simulink model "controller"  (Simulink 7.3)
settings: Solver=FixedStepDiscrete  StartTime=0.0  StopTime=inf  FixedStep=120  RelTol=1e-3
libraries: simulink x6
settings Model: Creator=mwetter  LastModifiedBy=mwetter

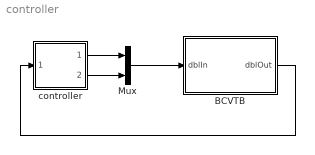
== system controller ==
  BCVTB : Subsystem  Description=Block that interfaces to the BCVTB.
  Mux : Mux  Inputs=2
  controller : Subsystem
  wires:
  controller/2(TSet) -> Mux/2
  controller/1(yHea) -> Mux/1
  Mux/1 -> BCVTB/1(dblIn)
  BCVTB/1(dblOut) -> controller/1(TMea)

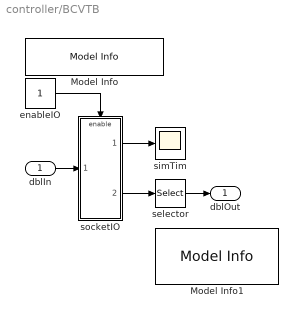
== system controller/BCVTB ==
  dblIn : Inport
  Model Info : simulink/Model-Wide Utilities/Model Info  SystemSampleTime=-1  InitialBlockCM=None  BlockCM=None  Frame=off  DisplayStringWithTags=%<Description>Set to 1 to enable I/O  HorizontalTextAlignment=Left  LeftAlignmentValue=0.02  SourceBlockDiagram=controller  TagMaxNumber=20
  Model Info1 : simulink/Model-Wide Utilities/Model Info  SystemSampleTime=-1  InitialBlockCM=None  BlockCM=None  Frame=off  DisplayStringWithTags=|  HorizontalTextAlignment=Left  LeftAlignmentValue=0.02  SourceBlockDiagram=controller  TagMaxNumber=20
      | The selector block selects 
      | a subset of the vector u 
      | and outputs it as the vector v.
  enableIO : Constant  OutDataType=sfix(16)  OutScaling=2^0
  selector : Selector  InputPortWidth=128  IndexOptions=Index vector (dialog)  Indices=[1]  OutputSizes=1
  simTim : Scope
  socketIO : Subsystem
  dblOut : Outport
  wires:
  selector/1 -> dblOut/1
  dblIn/1 -> socketIO/1(dblIn)
  socketIO/2(dblOut) -> selector/1
  enableIO/1 -> socketIO/Enable
  socketIO/1(simTim) -> simTim/1

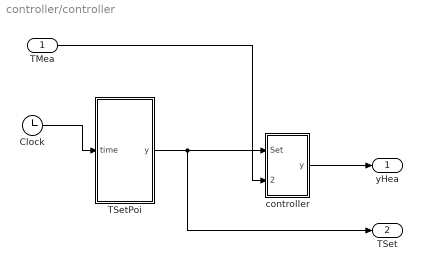
== system controller/controller ==
  TMea : Inport
  Clock : Clock
      settings: Decimation=10
  TSetPoi : Subsystem
  controller : Subsystem
  yHea : Outport
  TSet : Outport  Port=2
  wires:
  TSetPoi/1(y) -> controller/1(Set), TSet/1
  Clock/1 -> TSetPoi/1(time)
  TMea/1 -> controller/2(Mea)
  controller/1(y) -> yHea/1

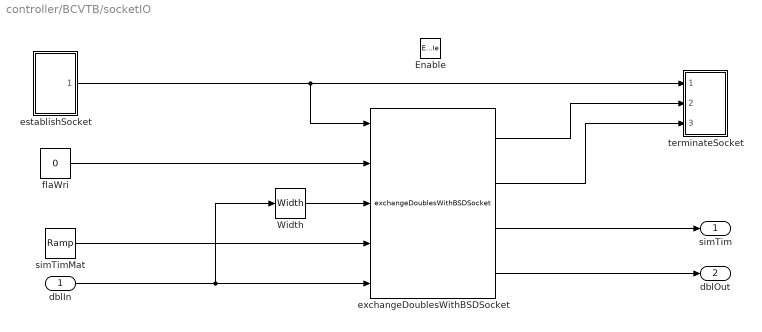
== system controller/BCVTB/socketIO ==
  dblIn : Inport
  Enable : EnablePort
  Width : Width  DataType=int16
  establishSocket : Subsystem  TreatAsAtomicUnit=on
  exchangeDoublesWithBSDSocket : S-Function  FunctionName=exchangeDoublesWithBSDSocket  EnableBusSupport=off  mask(Legacy Function){SFunctionSpec=int16 y1 = exchangeDoublesWithBSDSocket(int16 u1[1], int16 u2[1], int16 y2[1], double u3[1], double u4[], double y3[1], double y4[50]), ShowSpec=off}
      mask prompts: ShowSpec "Display function specification"
      mask help:
      | This block allows the user to call the following C function(s) in Simulink:
      |
      |  InitializeConditionsFcn: none
      |
      |  StartFcn: none
      |
      |  OutputFcn: int16 y1 = exchangeDoublesWithBSDSocket(int16 u1[1], int16 u2[1], int16 y2[1], double u3[1], double u4[], double y3[1], double y4[50])
      |
      |  TerminateFcn: none
      mask CallbackString:
      | |if strcmp(get_param(gcbh, 'ShowSpec'), 'on')
      |   set_param(gcbh, 'MaskDisplay', sprintf('fprintf(''%s'');', get_param(gcbh, 'SFunctionSpec')));
      | else
      |   set_param(gcbh, 'MaskDisplay', sprintf('fprintf(''%s'');', get_param(gcbh, 'FunctionName')));
      | end
      mask Display: fprintf('exchangeDoublesWithBSDSocket');
  flaWri : Constant  Value=0  OutDataTypeMode=int16  OutDataType=sfix(16)  OutScaling=2^0  OutDataTypeStr=int16
  simTimMat : simulink/Sources/Ramp  SystemSampleTime=-1  slope=1  start=0  X0=0
  terminateSocket : Subsystem
  simTim : Outport
  dblOut : Outport  Port=2
  wires:
  exchangeDoublesWithBSDSocket/2 -> terminateSocket/3(excFlaRea)
  exchangeDoublesWithBSDSocket/1 -> terminateSocket/2(excRetVal)
  exchangeDoublesWithBSDSocket/4 -> dblOut/1
  Width/1 -> exchangeDoublesWithBSDSocket/3
  simTimMat/1 -> exchangeDoublesWithBSDSocket/4
  dblIn/1 -> Width/1, exchangeDoublesWithBSDSocket/5
  exchangeDoublesWithBSDSocket/3 -> simTim/1
  flaWri/1 -> exchangeDoublesWithBSDSocket/2
  establishSocket/1(socketFD) -> terminateSocket/1(sockfd), exchangeDoublesWithBSDSocket/1

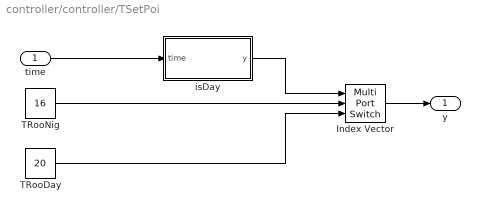
== system controller/controller/TSetPoi ==
  time : Inport  OutDataType=sfix(16)  OutScaling=2^0
  Index Vector : MultiPortSwitch  Inputs=2  zeroidx=on  OutDataType=sfix(16)  OutScaling=2^0
  TRooDay : Constant  Value=20  OutDataType=sfix(16)  OutScaling=2^0
  TRooNig : Constant  Value=16  OutDataType=sfix(16)  OutScaling=2^0
  isDay : Subsystem
  y : Outport  OutDataType=sfix(16)  OutScaling=2^0
  wires:
  time/1 -> isDay/1(time)
  Index Vector/1 -> y/1
  isDay/1(y) -> Index Vector/1
  TRooNig/1 -> Index Vector/2
  TRooDay/1 -> Index Vector/3

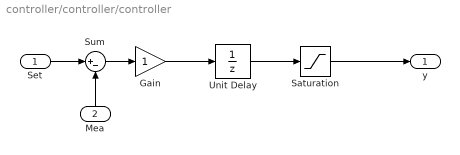
== system controller/controller/controller ==
  Set : Inport  OutDataType=sfix(16)  OutScaling=2^0
  Mea : Inport  Port=2
  Gain : Gain  ParameterDataType=sfix(16)  ParameterScaling=2^0  OutDataType=sfix(16)  OutScaling=2^0
  Saturation : Saturate  UpperLimit=1  LowerLimit=0  OutDataType=sfix(16)  OutScaling=2^0
  Sum : Sum  Inputs=|+-  OutDataType=sfix(16)  OutScaling=2^0
  Unit Delay : UnitDelay  SampleTime=-1
  y : Outport  OutDataType=sfix(16)  OutScaling=2^0
  wires:
  Set/1 -> Sum/1
  Sum/1 -> Gain/1
  Gain/1 -> Unit Delay/1
  Unit Delay/1 -> Saturation/1
  Mea/1 -> Sum/2
  Saturation/1 -> y/1

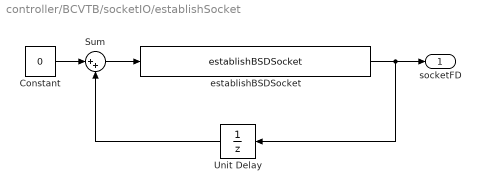
== system controller/BCVTB/socketIO/establishSocket ==
  Constant : Constant  Value=0  OutDataTypeMode=int16  OutDataType=sfix(16)  OutScaling=2^0  OutDataTypeStr=int16
  Sum : Sum  Inputs=|++  OutDataType=sfix(16)  OutScaling=2^0
  Unit Delay : UnitDelay  SampleTime=-1
  establishBSDSocket : S-Function  FunctionName=establishBSDSocket  EnableBusSupport=off  mask(Legacy Function){SFunctionSpec=int16 y1 = establishBSDSocket(int16 u1[1]), ShowSpec=on}
      mask prompts: ShowSpec "Display function specification"
      mask help:
      | This block allows the user to call the following C function(s) in Simulink:
      |
      |  InitializeConditionsFcn: none
      |
      |  StartFcn: none
      |
      |  OutputFcn: int16 y1 = establishBSDSocket(int16 u1[1])
      |
      |  TerminateFcn: none
      mask CallbackString:
      | |if strcmp(get_param(gcbh, 'ShowSpec'), 'on')
      |   set_param(gcbh, 'MaskDisplay', sprintf('fprintf(''%s'');', get_param(gcbh, 'SFunctionSpec')));
      | else
      |   set_param(gcbh, 'MaskDisplay', sprintf('fprintf(''%s'');', get_param(gcbh, 'FunctionName')));
      | end
      mask Display: fprintf('int16 y1 = establishBSDSocket(int16 u1[1])');
  socketFD : Outport
  wires:
  establishBSDSocket/1 -> Unit Delay/1, socketFD/1
  Sum/1 -> establishBSDSocket/1
  Constant/1 -> Sum/1
  Unit Delay/1 -> Sum/2

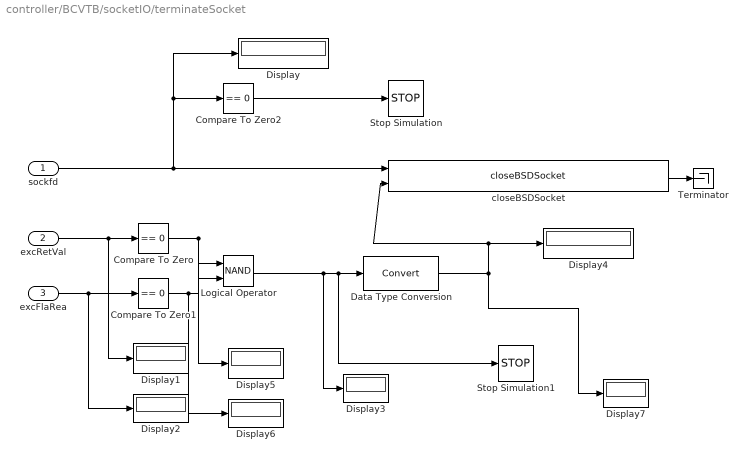
== system controller/BCVTB/socketIO/terminateSocket ==
  sockfd : Inport
  excRetVal : Inport  Port=2
  excFlaRea : Inport  Port=3
  Compare To Zero : simulink/Logic and Bit Operations/Compare To Zero  SystemSampleTime=-1  relop===  LogicOutDataTypeMode=uint8  ZeroCross=off
  Compare To Zero1 : simulink/Logic and Bit Operations/Compare To Zero  SystemSampleTime=-1  relop===  LogicOutDataTypeMode=uint8  ZeroCross=off
  Compare To Zero2 : simulink/Logic and Bit Operations/Compare To Zero  SystemSampleTime=-1  relop===  LogicOutDataTypeMode=boolean  ZeroCross=off
  Data Type Conversion : DataTypeConversion  OutDataType=sfix(16)  OutScaling=2^0
  Display{,1..7} (8 alike) : Display
  Logical Operator : Logic  Operator=NAND  AllPortsSameDT=off  OutDataTypeMode=boolean  OutDataTypeStr=boolean
  Stop Simulation : Stop
  Stop Simulation1 : Stop
  Terminator : Terminator
  closeBSDSocket : S-Function  FunctionName=closeBSDSocket  EnableBusSupport=off  mask(Legacy Function){SFunctionSpec=int16 y1 = closeBSDSocket(int16 u1[1], int16 u2[1]), ShowSpec=on}
      mask prompts: ShowSpec "Display function specification"
      mask help:
      | This block allows the user to call the following C function(s) in Simulink:
      |
      |  InitializeConditionsFcn: none
      |
      |  StartFcn: none
      |
      |  OutputFcn: int16 y1 = closeBSDSocket(int16 u1[1], int16 u2[1])
      |
      |  TerminateFcn: none
      mask CallbackString:
      | |if strcmp(get_param(gcbh, 'ShowSpec'), 'on')
      |   set_param(gcbh, 'MaskDisplay', sprintf('fprintf(''%s'');', get_param(gcbh, 'SFunctionSpec')));
      | else
      |   set_param(gcbh, 'MaskDisplay', sprintf('fprintf(''%s'');', get_param(gcbh, 'FunctionName')));
      | end
      mask Display: fprintf('int16 y1 = closeBSDSocket(int16 u1[1], int16 u2[1])');
  wires:
  closeBSDSocket/1 -> Terminator/1
  Compare To Zero2/1 -> Stop Simulation/1
  Data Type Conversion/1 -> Display7/1, Display4/1, closeBSDSocket/2
  Logical Operator/1 -> Stop Simulation1/1, Data Type Conversion/1, Display3/1
  Compare To Zero1/1 -> Display6/1, Logical Operator/2
  Compare To Zero/1 -> Display5/1, Logical Operator/1
  excFlaRea/1 -> Display2/1, Compare To Zero1/1
  excRetVal/1 -> Display1/1, Compare To Zero/1
  sockfd/1 -> Display/1, Compare To Zero2/1, closeBSDSocket/1

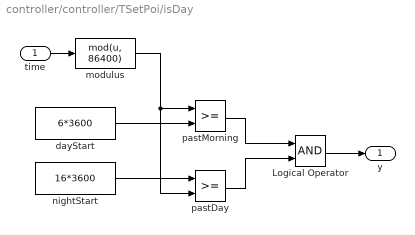
== system controller/controller/TSetPoi/isDay ==
  time : Inport
  Logical Operator : Logic  AllPortsSameDT=off  OutDataTypeMode=boolean  OutDataTypeStr=boolean
  dayStart : Constant  Value=6*3600  OutDataType=sfix(16)  OutScaling=2^0
  modulus : MATLABFcn  MATLABFcn=mod(u, 86400)
  nightStart : Constant  Value=16*3600  OutDataType=sfix(16)  OutScaling=2^0
  pastDay : RelationalOperator  LogicOutDataTypeMode=boolean  OutDataTypeStr=boolean
  pastMorning : RelationalOperator  LogicOutDataTypeMode=boolean  OutDataTypeStr=boolean
  y : Outport
  wires:
  time/1 -> modulus/1
  modulus/1 -> pastMorning/1, pastDay/2
  dayStart/1 -> pastMorning/2
  nightStart/1 -> pastDay/1
  pastMorning/1 -> Logical Operator/1
  pastDay/1 -> Logical Operator/2
  Logical Operator/1 -> y/1
